simulink model "robot_forward_kinematics"  (R2019b)
settings: Solver=VariableStepAuto  StartTime=0.0  StopTime=10.0  RelTol=1e-3
libraries: simulink_extras x2
settings Model: Creator=Davide  LastModifiedBy=Davide

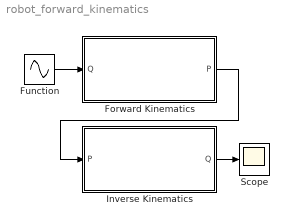
== system robot_forward_kinematics ==
  " Scope" : Scope
  Forward Kinematics : Subsystem
  Function : Sin  SampleTime=0
  Inverse Kinematics : Subsystem
  wires:
  Function/1 -> Forward Kinematics/1(Q)
  Forward Kinematics/1(P) -> Inverse Kinematics/1(P)
  Inverse Kinematics/1(Q) -> " Scope"/1

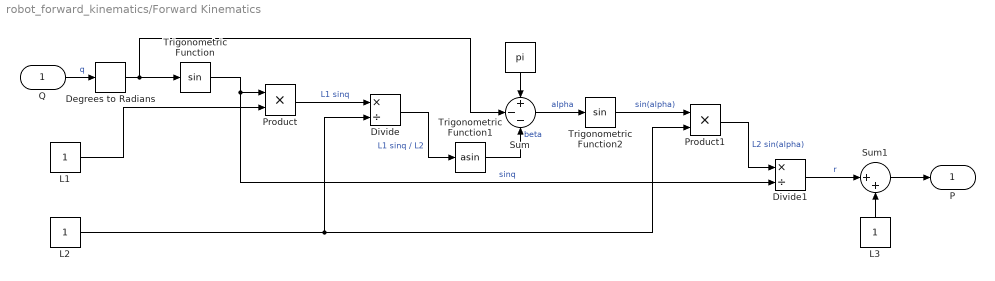
== system robot_forward_kinematics/Forward Kinematics ==
  Q : Inport
  " " : Constant  Value=pi
  Degrees to Radians : simulink_extras/Transformations/Degrees to Radians
  Divide : Product  Inputs=*/
  Divide1 : Product  Inputs=*/
  L1 : Constant
  L2 : Constant
  L3 : Constant
  Product : Product
  Product1 : Product
  Sum : Sum  Inputs=+--
  Sum1 : Sum  Inputs=|++
  Trigonometric Function : Trigonometry
  Trigonometric Function1 : Trigonometry  Operator=asin
  Trigonometric Function2 : Trigonometry
  P : Outport
  wires:
  Trigonometric Function/1 -> Product/1, Divide1/2  "sinq"
  L1/1 -> Product/2
  Product/1 -> Divide/1  "L1 sinq"
  L2/1 -> Product1/2, Divide/2
  Divide/1 -> Trigonometric Function1/1  "L1 sinq / L2"
  " "/1 -> Sum/1
  Trigonometric Function1/1 -> Sum/3  "beta"
  Sum/1 -> Trigonometric Function2/1  "alpha"
  Trigonometric Function2/1 -> Product1/1  "sin(alpha)"
  Product1/1 -> Divide1/1  "L2 sin(alpha)"
  Divide1/1 -> Sum1/1  "r"
  L3/1 -> Sum1/2
  Sum1/1 -> P/1
  Q/1 -> Degrees to Radians/1  "q"
  Degrees to Radians/1 -> Sum/2, Trigonometric Function/1

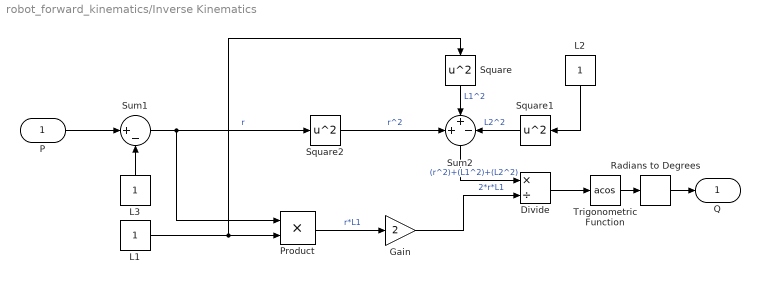
== system robot_forward_kinematics/Inverse Kinematics ==
  P : Inport
  Divide : Product  Inputs=*/
  Gain : Gain  Gain=2
  L1 : Constant
  L2 : Constant
  L3 : Constant
  Product : Product
  Radians to Degrees : simulink_extras/Transformations/Radians to Degrees
  Square : Math  Operator=square  SignedPower=off  SaturateOnIntegerOverflow=on
  Square1 : Math  Operator=square  SignedPower=off  SaturateOnIntegerOverflow=on
  Square2 : Math  Operator=square  SignedPower=off  SaturateOnIntegerOverflow=on
  Sum1 : Sum  Inputs=|+-
  Sum2 : Sum  Inputs=++-
  Trigonometric Function : Trigonometry  Operator=acos
  Q : Outport
  wires:
  P/1 -> Sum1/1
  L3/1 -> Sum1/2
  Divide/1 -> Trigonometric Function/1
  Product/1 -> Gain/1  "r*L1"
  Gain/1 -> Divide/2  "2*r*L1"
  Sum1/1 -> Square2/1, Product/1  "r"
  L1/1 -> Product/2, Square/1
  Sum2/1 -> Divide/1  "(r^2)+(L1^2)+(L2^2)"
  Square2/1 -> Sum2/1  "r^2"
  L2/1 -> Square1/1
  Square1/1 -> Sum2/3  "L2^2"
  Square/1 -> Sum2/2  "L1^2"
  Trigonometric Function/1 -> Radians to Degrees/1
  Radians to Degrees/1 -> Q/1
